simulink model "Test_Counter_4bit"  (R2016a)
settings: Solver=VariableStepAuto  StartTime=0.0  StopTime=1000.0  MaxStep=1  MinStep=1  RelTol=1e-3
libraries: commutil2 x1, simulink_extras x1, Clock_Lib x1
settings Model: PauseTimes=0  Creator=Jozko Mrkvicka  LastModifiedBy=Jozko Mrkvicka
settings SolverCC: InitialStep=1

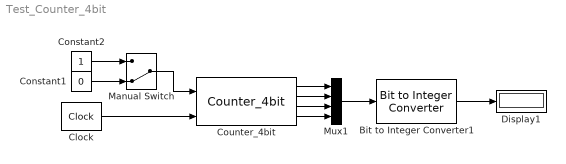
== system Test_Counter_4bit ==
  Bit to Integer Converter1 : commutil2/Bit to Integer Converter  nbits=4  bitOrder=MSB first  signedOutputValues=Unsigned  outDtype=uint8  outDtypeSigned=Inherit via internal rule
  Clock : simulink_extras/Flip Flops/Clock  period=2
  Constant1 : Constant  Value=0
  Constant2 : Constant
  Counter_4bit : Clock_Lib/Counter_4bit
  Display1 : Display
  Manual Switch : ManualSwitch  CurrentSetting=0
  Mux1 : Mux
  wires:
  Clock/1 -> Counter_4bit/2
  Counter_4bit/1 -> Mux1/1
  Counter_4bit/3 -> Mux1/3
  Mux1/1 -> Bit to Integer Converter1/1
  Bit to Integer Converter1/1 -> Display1/1
  Manual Switch/1 -> Counter_4bit/1
  Counter_4bit/2 -> Mux1/2
  Constant2/1 -> Manual Switch/1
  Constant1/1 -> Manual Switch/2
  Counter_4bit/4 -> Mux1/4
